simulink model "FFM_Punch"  (R2017a)
settings: Solver=ode3  StartTime=0.0  StopTime=timesteps  FixedStep=data.SIM.Ts  RelTol=1e-3  EnableMultiTasking=on
values from neighbouring files (symbols this model uses):
  data =     [dakota_config.mat]
  downshift_map = data.TCU.upshift.veh_spd_default    [Simulation_results.m]
  upshift_map = data.TCU.upshift.veh_spd_default    [Simulation_results.m]
undefined symbols (not defined in the file or in its folder): air_density, Cd, DiscIntNeverNeededParam, fr_crankshaft, fr_speed_values, g, i_FD, ICE, Low_Ratio, M_Eng_Max, M_Eng_Max_Max, M_Eng_Max_Rpm, mt2m_f, mu_Roll_C0, mu_Roll_C1, mu_Roll_C2, Mv, n_Idle_Eng, Overdrive_Ratio, Re, S_eff_drag, Ts
(part 7 of 15)

== system FFM_Punch/Driver Interface/Driver Model-_old/Rolling Resistance ==
  v_Ref : Inport
  Fcn1 : Fcn  Expr=u(1)*(u(2)+u(3)*u(8)+u(4)*u(8)*u(8)+u(5)*u(8)*u(8)*u(8)+u(6)*u(8)*u(8)*u(8)*u(8)+u(7)*u(8)*u(8)*u(8)*u(8)*u(8))
  Lookup Table : Lookup  InputValues=[-1e3 -1 0 1 1e3 ]  Table=[1 1 0 -1 -1]  LookUpMeth=Interpolation-Use End Values
  Mux1 : Mux  Inputs=8
  Product : Product  RndMeth=Zero
  Roll_res_coeff_C2 : Constant  Value=Mv*g
  Roll_res_coeff_C3 : Constant  Value=mu_Roll_C0
  Roll_res_coeff_C4 : Constant  Value=mu_Roll_C1
  Roll_res_coeff_C5 : Constant  Value=mu_Roll_C2
  Roll_res_coeff_C6 : Constant  Value=0
  kph2m/sec : Gain  Gain=1/3.6  OutDataTypeStr=Inherit: Inherit via back propagation  ParamDataTypeStr=Inherit: Same as input
  mu_Roll_C4 : Constant  Value=0
  mu_Roll_C5 : Constant  Value=0
  radius tyre : Gain  Gain=-Re  OutDataTypeStr=Inherit: Inherit via back propagation  ParamDataTypeStr=Inherit: Same as input
  M_RollingRes : Outport
  wires:
  mu_Roll_C5/1 -> Mux1/7
  kph2m/sec/1 -> Mux1/8
  mu_Roll_C4/1 -> Mux1/6
  Roll_res_coeff_C6/1 -> Mux1/5
  Roll_res_coeff_C5/1 -> Mux1/4
  Product/1 -> M_RollingRes/1
  v_Ref/1 -> kph2m/sec/1, Lookup Table/1
  radius tyre/1 -> Product/1
  Roll_res_coeff_C2/1 -> Mux1/1
  Fcn1/1 -> radius tyre/1
  Roll_res_coeff_C4/1 -> Mux1/3
  Roll_res_coeff_C3/1 -> Mux1/2
  Mux1/1 -> Fcn1/1
  Lookup Table/1 -> Product/2

== system FFM_Punch/Driver Interface/Driver Model-_old/Signed square ==
  note: Air Density
  Vehicle Speed : Inport
  Drag Coefficient : Gain  Gain=Cd  OutDataTypeStr=Inherit: Inherit via back propagation  ParamDataTypeStr=Inherit: Same as input
  Frontal Area : Gain  Gain=S_eff_drag  OutDataTypeStr=Inherit: Inherit via back propagation  ParamDataTypeStr=Inherit: Same as input
  Gain3 : Gain  Gain=0.5
  Product : Product  Inputs=3  RndMeth=Zero
  Sign : Signum  ZeroCross=off
  rho : Gain  Gain=air_density
  Aerodynamic Drag Force : Outport
  wires:
  Sign/1 -> Product/3
  Product/1 -> rho/1
  Gain3/1 -> Aerodynamic Drag Force/1
  Frontal Area/1 -> Gain3/1
  Drag Coefficient/1 -> Frontal Area/1
  rho/1 -> Drag Coefficient/1
  Vehicle Speed/1 -> Product/1, Product/2, Sign/1

== system FFM_Punch/Vehicle/Subsystem/Rolling Resistance ==
  v_veh : Inport
  Abs : Abs
  Constant : Constant  Tag=Controls_Lib  Description=constant  Value=Value  OutMin=OutMin  OutMax=OutMax  OutDataTypeStr=Inherit: Inherit via back propagation  SampleTime=SampleTime  FramePeriod=FramePeriod  mask(Constant){Value=1, VectorParams1D=on, SampleTime=-1, FramePeriod=inf, OutMin=[], OutMax=[], OutDataTypeStr=Inherit: Inherit via back propagation, LockScale=off}
      mask prompts: Value "Simulink:blkprm_prompts:ConstConstValue"; VectorParams1D "Simulink:blkprm_prompts:AllSrcsVector1D"; SampleTime "Simulink:blkprm_prompts:AllSrcBlksSampleTime"; FramePeriod "Simulink:blkprm_prompts:AllSrcBlksFramePeriod"; OutMin "Simulink:blkprm_prompts:OutputDesignMin"; OutMax "Simulink:blkprm_prompts:OutputDesignMax"; OutDataTypeStr "Simulink:blkprm_prompts:OUTPUT_UNIFIEDDATATYPE"; LockScale "Simulink:blkprm_prompts:LockScale"
      mask help: Output the constant specified by the 'Constant value' parameter.
      mask Help: web([fileparts(which('Lib_built')) filesep 'hlp' filesep 'lib_constant' '.html'], '-helpbrowser')
      mask TypeOptions Value: Value
      mask TypeOptions VectorParams1D: VectorParams1D
      mask TypeOptions SampleTime: SampleTime
      mask TypeOptions FramePeriod: FramePeriod
      mask TypeOptions OutMin: OutMin
      mask TypeOptions OutMax: OutMax
      mask TypeOptions OutDataTypeStr: OutDataTypeStr
      mask TypeOptions LockScale: LockScale
      mask DialogControl ParameterTabVar0 Prompt: Main
      mask Display: disp(get_param(gcb,'Value'))
  Constant1 : Constant  Tag=Controls_Lib  Description=constant  Value=Value  OutMin=OutMin  OutMax=OutMax  OutDataTypeStr=Inherit: Inherit via back propagation  SampleTime=SampleTime  FramePeriod=FramePeriod  mask(Constant){Value=0, VectorParams1D=on, SampleTime=-1, FramePeriod=inf, OutMin=[], OutMax=[], OutDataTypeStr=Inherit: Inherit via back propagation, LockScale=off}
      mask prompts: Value "Simulink:blkprm_prompts:ConstConstValue"; VectorParams1D "Simulink:blkprm_prompts:AllSrcsVector1D"; SampleTime "Simulink:blkprm_prompts:AllSrcBlksSampleTime"; FramePeriod "Simulink:blkprm_prompts:AllSrcBlksFramePeriod"; OutMin "Simulink:blkprm_prompts:OutputDesignMin"; OutMax "Simulink:blkprm_prompts:OutputDesignMax"; OutDataTypeStr "Simulink:blkprm_prompts:OUTPUT_UNIFIEDDATATYPE"; LockScale "Simulink:blkprm_prompts:LockScale"
      mask help: Output the constant specified by the 'Constant value' parameter.
      mask Help: web([fileparts(which('Lib_built')) filesep 'hlp' filesep 'lib_constant' '.html'], '-helpbrowser')
      mask TypeOptions Value: Value
      mask TypeOptions VectorParams1D: VectorParams1D
      mask TypeOptions SampleTime: SampleTime
      mask TypeOptions FramePeriod: FramePeriod
      mask TypeOptions OutMin: OutMin
      mask TypeOptions OutMax: OutMax
      mask TypeOptions OutDataTypeStr: OutDataTypeStr
      mask TypeOptions LockScale: LockScale
      mask DialogControl ParameterTabVar0 Prompt: Main
      mask Display: disp(get_param(gcb,'Value'))
  Convert : DataTypeConversion  Tag=Controls_Lib  Description=Convert  OutMin=OutMin  OutMax=OutMax  RndMeth=Round  SampleTime=SampleTime  SaturateOnIntegerOverflow=on  mask(Datatype conversion){ConvertRealWorld=Real World Value (RWV), SampleTime=-1, OutMin=[], OutMax=[], OutDataTypeStr=Inherit: Inherit via back propagation, LockScale=off, RndMeth=Round, SaturateOnIntegerOverflow=on}
      mask prompts: ConvertRealWorld "Input and output to have equal:"; SampleTime "Sample time (-1 for inherited):"; OutMin "Output minimum:"; OutMax "Output maximum:"; OutDataTypeStr "Output data type:"; LockScale "Lock output data type setting against changes by the fixed-point tools"; RndMeth "Integer rounding mode:"; SaturateOnIntegerOverflow "Saturate on integer overflow"
      mask help: Convert the input to the data type and scaling of the output.
      mask Help: web([fileparts(which('Lib_built')) filesep 'hlp' filesep 'lib_DataTypeConv' '.html'], '-helpbrowser')
      mask TypeOptions ConvertRealWorld: ConvertRealWorld
      mask TypeOptions SampleTime: SampleTime
      mask TypeOptions OutMin: OutMin
      mask TypeOptions OutMax: OutMax
      mask TypeOptions OutDataTypeStr: OutDataTypeStr
      mask TypeOptions LockScale: LockScale
      mask TypeOptions RndMeth: RndMeth
      mask TypeOptions SaturateOnIntegerOverflow: SaturateOnIntegerOverflow
  Fcn : Fcn  Expr=u(1)*(u(2)+u(3)*u(8)+u(4)*u(8)*u(8)+u(5)*u(8)*u(8)*u(8)+u(6)*u(8)*u(8)*u(8)*u(8)+u(7)*u(8)*u(8)*u(8)*u(8)*u(8))
  Mux1 : Mux  Inputs=8
  Roll_res_coeff_C0 : Constant  Value=data.VEH.mu_Roll_C0
  Roll_res_coeff_C1 : Constant  Value=data.VEH.mu_Roll_C1
  Roll_res_coeff_C2 : Constant  Value=data.VEH.mu_Roll_C2
  Roll_res_coeff_C3 : Constant  Value=data.VEH.mu_Roll_C3
  Switch : Switch  Criteria=u2 > Threshold  Threshold=eps
  "Weight Vehicle " : Gain  Gain=data.VEH.Mv*data.VEH.g  OutDataTypeStr=Inherit: Inherit via back propagation  ParamDataTypeStr=Inherit: Same as input
  mu_Roll_C4 : Constant  Value=data.VEH.mu_Roll_C4
  mu_Roll_C5 : Constant  Value=data.VEH.mu_Roll_C5
  F_RR : Outport  Tag=Controls_Lib  Description=Out  InitialOutput=0
  wires:
  Abs/1 -> Mux1/8
  mu_Roll_C5/1 -> Mux1/7
  mu_Roll_C4/1 -> Mux1/6
  Roll_res_coeff_C3/1 -> Mux1/5
  Roll_res_coeff_C2/1 -> Mux1/4
  v_veh/1 -> Switch/2, Abs/1
  Roll_res_coeff_C1/1 -> Mux1/3
  Roll_res_coeff_C0/1 -> Mux1/2
  Mux1/1 -> Fcn/1
  "Weight Vehicle "/1 -> Mux1/1
  Constant/1 -> "Weight Vehicle "/1
  Fcn/1 -> Convert/1
  Constant1/1 -> Switch/3
  Switch/1 -> F_RR/1
  Convert/1 -> Switch/1

== system FFM_Punch/Vehicle/Subsystem/Signed square ==
  note: Air Density
  Vehicle Speed : Inport
  Convert : DataTypeConversion  Tag=Controls_Lib  Description=Convert  OutMin=OutMin  OutMax=OutMax  RndMeth=Round  SampleTime=SampleTime  SaturateOnIntegerOverflow=on  mask(Datatype conversion){ConvertRealWorld=Real World Value (RWV), SampleTime=-1, OutMin=[], OutMax=[], OutDataTypeStr=Inherit: Inherit via back propagation, LockScale=off, RndMeth=Round, SaturateOnIntegerOverflow=on}
      mask prompts: ConvertRealWorld "Input and output to have equal:"; SampleTime "Sample time (-1 for inherited):"; OutMin "Output minimum:"; OutMax "Output maximum:"; OutDataTypeStr "Output data type:"; LockScale "Lock output data type setting against changes by the fixed-point tools"; RndMeth "Integer rounding mode:"; SaturateOnIntegerOverflow "Saturate on integer overflow"
      mask help: Convert the input to the data type and scaling of the output.
      mask Help: web([fileparts(which('Lib_built')) filesep 'hlp' filesep 'lib_DataTypeConv' '.html'], '-helpbrowser')
      mask TypeOptions ConvertRealWorld: ConvertRealWorld
      mask TypeOptions SampleTime: SampleTime
      mask TypeOptions OutMin: OutMin
      mask TypeOptions OutMax: OutMax
      mask TypeOptions OutDataTypeStr: OutDataTypeStr
      mask TypeOptions LockScale: LockScale
      mask TypeOptions RndMeth: RndMeth
      mask TypeOptions SaturateOnIntegerOverflow: SaturateOnIntegerOverflow
  Drag Coefficient : Gain  Gain=data.VEH.Cd  OutDataTypeStr=Inherit: Inherit via back propagation  ParamDataTypeStr=Inherit: Same as input
  Frontal Area : Gain  Gain=data.VEH.S_eff_drag  OutDataTypeStr=Inherit: Inherit via back propagation  ParamDataTypeStr=Inherit: Same as input
  Gain3 : Gain  Gain=0.5
  Product : Product  RndMeth=Zero
  Product1 : Product  RndMeth=Zero
  Sign : Signum  ZeroCross=off
  rho : Gain  Gain=data.VEH.air_density
  Aerodynamic Drag Force : Outport
  wires:
  Sign/1 -> Product/2
  Frontal Area/1 -> Gain3/1
  Drag Coefficient/1 -> Frontal Area/1
  rho/1 -> Drag Coefficient/1
  Product/1 -> rho/1
  Vehicle Speed/1 -> Product1/2, Product1/1, Sign/1
  Product1/1 -> Product/1
  Gain3/1 -> Convert/1
  Convert/1 -> Aerodynamic Drag Force/1

== system FFM_Punch/Controller/F02_03_03_05_Raw_Gear_Target_Auto_Mode/F02_03_03_05_09_Final_Raw_Gear_Target_Auto_Mode/TurnOnDelay1 ==
  b_Input : Inport  Tag=Controls_Lib  Description=Inp  OutDataTypeStr=boolean  Interpolate=off
  Tdly : Inport  Tag=Controls_Lib  Description=Inp  Port=2  OutDataTypeStr=single  Interpolate=off
  Constant2 : Constant  Tag=Controls_Lib  Description=constant  Value=Value  OutMin=OutMin  OutMax=OutMax  OutDataTypeStr=boolean  SampleTime=SampleTime  FramePeriod=FramePeriod  mask(Constant){Value=0, VectorParams1D=on, SampleTime=-1, FramePeriod=inf, OutMin=[], OutMax=[], OutDataTypeStr=boolean, LockScale=off}
      mask prompts: Value "Simulink:blkprm_prompts:ConstConstValue"; VectorParams1D "Simulink:blkprm_prompts:AllSrcsVector1D"; SampleTime "Simulink:blkprm_prompts:AllSrcBlksSampleTime"; FramePeriod "Simulink:blkprm_prompts:AllSrcBlksFramePeriod"; OutMin "Simulink:blkprm_prompts:OutputDesignMin"; OutMax "Simulink:blkprm_prompts:OutputDesignMax"; OutDataTypeStr "Simulink:blkprm_prompts:OUTPUT_UNIFIEDDATATYPE"; LockScale "Simulink:blkprm_prompts:LockScale"
      mask help: Output the constant specified by the 'Constant value' parameter.
      mask Help: web([fileparts(which('Lib_built')) filesep 'hlp' filesep 'lib_constant' '.html'], '-helpbrowser')
      mask TypeOptions Value: Value
      mask TypeOptions VectorParams1D: VectorParams1D
      mask TypeOptions SampleTime: SampleTime
      mask TypeOptions FramePeriod: FramePeriod
      mask TypeOptions OutMin: OutMin
      mask TypeOptions OutMax: OutMax
      mask TypeOptions OutDataTypeStr: OutDataTypeStr
      mask TypeOptions LockScale: LockScale
      mask DialogControl ParameterTabVar0 Prompt: Main
      mask Display: disp(get_param(gcb,'Value'))
  Logic : Logic  Tag=Controls_Lib  Description=Logic  Operator=NOT  Inputs=Inputs  OutDataTypeStr=boolean  SampleTime=SampleTime  mask(Logic){Operator=NOT, Inputs=2, IconShape=rectangular, SampleTime=-1, AllPortsSameDT=on, OutDataTypeStr=boolean}
      mask prompts: Inputs "Number of input ports:"; IconShape "Icon shape:"; SampleTime "Sample time (-1 for inherited):"; AllPortsSameDT "Require all inputs and output to have the same data type"; OutDataTypeStr "Output data type:"
      mask help: Logical operators. For a single input, operators are applied across the input vector. For multiple inputs, operators are applied across the inputs.
      mask Help: web([fileparts(which('Lib_built')) filesep 'hlp' filesep 'lib_Logic' '.html'], '-helpbrowser')
      mask TypeOptions Operator: Operator
      mask TypeOptions Inputs: Inputs
      mask TypeOptions IconShape: IconShape
      mask TypeOptions SampleTime: SampleTime
      mask TypeOptions AllPortsSameDT: AllPortsSameDT
      mask TypeOptions OutDataTypeStr: OutDataTypeStr
  Logic1 : Logic  Tag=Controls_Lib  Description=Logic  Operator=NOT  Inputs=Inputs  OutDataTypeStr=boolean  SampleTime=SampleTime  mask(Logic){Operator=NOT, Inputs=2, IconShape=rectangular, SampleTime=-1, AllPortsSameDT=on, OutDataTypeStr=boolean}
      mask prompts: Inputs "Number of input ports:"; IconShape "Icon shape:"; SampleTime "Sample time (-1 for inherited):"; AllPortsSameDT "Require all inputs and output to have the same data type"; OutDataTypeStr "Output data type:"
      mask help: Logical operators. For a single input, operators are applied across the input vector. For multiple inputs, operators are applied across the inputs.
      mask Help: web([fileparts(which('Lib_built')) filesep 'hlp' filesep 'lib_Logic' '.html'], '-helpbrowser')
      mask TypeOptions Operator: Operator
      mask TypeOptions Inputs: Inputs
      mask TypeOptions IconShape: IconShape
      mask TypeOptions SampleTime: SampleTime
      mask TypeOptions AllPortsSameDT: AllPortsSameDT
      mask TypeOptions OutDataTypeStr: OutDataTypeStr
  Rising_Edge_DetectChange1 : Subsystem  Tag=Controls_Lib  Description=DetectChange  mask(Rising_Edge_Detect_change){}
      mask help:
      | Rising Edge Detect change block will detect the change in input signal.The block output will be true for one sample when input chnage from false to true.
      |
      | Note: Input and initial conditions must always be a boolean. Initial condition is used to enable or disable the edge detection at the very first instant. No Edge will be detected at the first instant if the Initial condition is set to be equal to the Input signal.
      mask init:
      | x1=[1 2 2 4 4 5];
      | y1=[7 7 9 9 9 9];
      | x2=[1 2 2 4 4 5];
      | y2=[0 0 0 0 0 0];
      mask Help: web([fileparts(which('Lib_discontious')) filesep 'hlp' filesep 'lib_DetectChange.html'], '-helpbrowser')
      mask Display: plot(x1,y1);plot(x2,y2);
  Terminator1 : Terminator
      settings: Tag=Controls_Lib  Description=Terminator
  Timer : Subsystem  Tag=Controls_Lib  Description=Timer  mask(Timer){}
      mask help:
      | This block counts down from TT to 0 (zero) when a falling edge is detected in the the 'Res' port. When the timer is active and 'Res' is FALSE, 'TL' specifies the time left to reach 0(zero). When 'Res' is TRUE, TL=TT. The output 'Busy' is TRUE when 'Res' TRUE or the timer is actively counting(i.e until 'TL' is 0(zero) ).
      |
      | Ports:
      | TT - Target Time [sec] [Single]
      | Res - Reset [-] [Boolean]
      | Busy - Busy status [-] [Boolean]
      | TL - Time Left [Sec] [Single]
      |
      | Input Guidelines:
      |
      | 1.The input 'TT' must always be a positive non-zero number.
      | 2.The input 'TT' must be a multiple of the fundamental sample time of the block.
      settings: RTWSystemCode=Inline
      mask Help: web([fileparts(which('Lib_math_logic')) filesep 'hlp' filesep 'lib_Timer.html'], '-helpbrowser')
      mask Display:
      | disp('Timer');
      | port_label('Input',1,'Res');
      | port_label('Input',2,'TT [s]');
      | port_label('Output',1,'Busy');
      | port_label('Output',2,'TL [s]');
  b_Output : Outport  OutDataTypeStr=boolean  OutputWhenDisabled=reset  InitialOutput=0
  wires:
  Timer/2(TL) -> Terminator1/1
  Timer/1(Busy) -> Logic1/1
  Logic/1 -> Timer/1(Res)
  b_Input/1 -> Logic/1
  Tdly/1 -> Timer/2(TT)
  Logic1/1 -> Rising_Edge_DetectChange1/1(b_Input)
  Rising_Edge_DetectChange1/1(b_Output) -> b_Output/1
  Constant2/1 -> Rising_Edge_DetectChange1/2(b_InitialValue)

== system FFM_Punch/Controller/F02_03_03_05_Raw_Gear_Target_Auto_Mode/F02_03_03_05_09_Final_Raw_Gear_Target_Auto_Mode/TurnOnDelay2 ==
  b_Input : Inport  Tag=Controls_Lib  Description=Inp  OutDataTypeStr=boolean  Interpolate=off
  Tdly : Inport  Tag=Controls_Lib  Description=Inp  Port=2  OutDataTypeStr=single  Interpolate=off
  Constant2 : Constant  Tag=Controls_Lib  Description=constant  Value=Value  OutMin=OutMin  OutMax=OutMax  OutDataTypeStr=boolean  SampleTime=SampleTime  FramePeriod=FramePeriod  mask(Constant){Value=0, VectorParams1D=on, SampleTime=-1, FramePeriod=inf, OutMin=[], OutMax=[], OutDataTypeStr=boolean, LockScale=off}
      mask prompts: Value "Simulink:blkprm_prompts:ConstConstValue"; VectorParams1D "Simulink:blkprm_prompts:AllSrcsVector1D"; SampleTime "Simulink:blkprm_prompts:AllSrcBlksSampleTime"; FramePeriod "Simulink:blkprm_prompts:AllSrcBlksFramePeriod"; OutMin "Simulink:blkprm_prompts:OutputDesignMin"; OutMax "Simulink:blkprm_prompts:OutputDesignMax"; OutDataTypeStr "Simulink:blkprm_prompts:OUTPUT_UNIFIEDDATATYPE"; LockScale "Simulink:blkprm_prompts:LockScale"
      mask help: Output the constant specified by the 'Constant value' parameter.
      mask Help: web([fileparts(which('Lib_built')) filesep 'hlp' filesep 'lib_constant' '.html'], '-helpbrowser')
      mask TypeOptions Value: Value
      mask TypeOptions VectorParams1D: VectorParams1D
      mask TypeOptions SampleTime: SampleTime
      mask TypeOptions FramePeriod: FramePeriod
      mask TypeOptions OutMin: OutMin
      mask TypeOptions OutMax: OutMax
      mask TypeOptions OutDataTypeStr: OutDataTypeStr
      mask TypeOptions LockScale: LockScale
      mask DialogControl ParameterTabVar0 Prompt: Main
      mask Display: disp(get_param(gcb,'Value'))
  Logic : Logic  Tag=Controls_Lib  Description=Logic  Operator=NOT  Inputs=Inputs  OutDataTypeStr=boolean  SampleTime=SampleTime  mask(Logic){Operator=NOT, Inputs=2, IconShape=rectangular, SampleTime=-1, AllPortsSameDT=on, OutDataTypeStr=boolean}
      mask prompts: Inputs "Number of input ports:"; IconShape "Icon shape:"; SampleTime "Sample time (-1 for inherited):"; AllPortsSameDT "Require all inputs and output to have the same data type"; OutDataTypeStr "Output data type:"
      mask help: Logical operators. For a single input, operators are applied across the input vector. For multiple inputs, operators are applied across the inputs.
      mask Help: web([fileparts(which('Lib_built')) filesep 'hlp' filesep 'lib_Logic' '.html'], '-helpbrowser')
      mask TypeOptions Operator: Operator
      mask TypeOptions Inputs: Inputs
      mask TypeOptions IconShape: IconShape
      mask TypeOptions SampleTime: SampleTime
      mask TypeOptions AllPortsSameDT: AllPortsSameDT
      mask TypeOptions OutDataTypeStr: OutDataTypeStr
  Logic1 : Logic  Tag=Controls_Lib  Description=Logic  Operator=NOT  Inputs=Inputs  OutDataTypeStr=boolean  SampleTime=SampleTime  mask(Logic){Operator=NOT, Inputs=2, IconShape=rectangular, SampleTime=-1, AllPortsSameDT=on, OutDataTypeStr=boolean}
      mask prompts: Inputs "Number of input ports:"; IconShape "Icon shape:"; SampleTime "Sample time (-1 for inherited):"; AllPortsSameDT "Require all inputs and output to have the same data type"; OutDataTypeStr "Output data type:"
      mask help: Logical operators. For a single input, operators are applied across the input vector. For multiple inputs, operators are applied across the inputs.
      mask Help: web([fileparts(which('Lib_built')) filesep 'hlp' filesep 'lib_Logic' '.html'], '-helpbrowser')
      mask TypeOptions Operator: Operator
      mask TypeOptions Inputs: Inputs
      mask TypeOptions IconShape: IconShape
      mask TypeOptions SampleTime: SampleTime
      mask TypeOptions AllPortsSameDT: AllPortsSameDT
      mask TypeOptions OutDataTypeStr: OutDataTypeStr
  Rising_Edge_DetectChange1 : Subsystem  Tag=Controls_Lib  Description=DetectChange  mask(Rising_Edge_Detect_change){}
      mask help:
      | Rising Edge Detect change block will detect the change in input signal.The block output will be true for one sample when input chnage from false to true.
      |
      | Note: Input and initial conditions must always be a boolean. Initial condition is used to enable or disable the edge detection at the very first instant. No Edge will be detected at the first instant if the Initial condition is set to be equal to the Input signal.
      mask init:
      | x1=[1 2 2 4 4 5];
      | y1=[7 7 9 9 9 9];
      | x2=[1 2 2 4 4 5];
      | y2=[0 0 0 0 0 0];
      mask Help: web([fileparts(which('Lib_discontious')) filesep 'hlp' filesep 'lib_DetectChange.html'], '-helpbrowser')
      mask Display: plot(x1,y1);plot(x2,y2);
  Terminator1 : Terminator
      settings: Tag=Controls_Lib  Description=Terminator
  Timer : Subsystem  Tag=Controls_Lib  Description=Timer  mask(Timer){}
      mask help:
      | This block counts down from TT to 0 (zero) when a falling edge is detected in the the 'Res' port. When the timer is active and 'Res' is FALSE, 'TL' specifies the time left to reach 0(zero). When 'Res' is TRUE, TL=TT. The output 'Busy' is TRUE when 'Res' TRUE or the timer is actively counting(i.e until 'TL' is 0(zero) ).
      |
      | Ports:
      | TT - Target Time [sec] [Single]
      | Res - Reset [-] [Boolean]
      | Busy - Busy status [-] [Boolean]
      | TL - Time Left [Sec] [Single]
      |
      | Input Guidelines:
      |
      | 1.The input 'TT' must always be a positive non-zero number.
      | 2.The input 'TT' must be a multiple of the fundamental sample time of the block.
      settings: RTWSystemCode=Inline
      mask Help: web([fileparts(which('Lib_math_logic')) filesep 'hlp' filesep 'lib_Timer.html'], '-helpbrowser')
      mask Display:
      | disp('Timer');
      | port_label('Input',1,'Res');
      | port_label('Input',2,'TT [s]');
      | port_label('Output',1,'Busy');
      | port_label('Output',2,'TL [s]');
  b_Output : Outport  OutDataTypeStr=boolean  OutputWhenDisabled=reset  InitialOutput=0
  wires:
  Constant2/1 -> Rising_Edge_DetectChange1/2(b_InitialValue)
  Rising_Edge_DetectChange1/1(b_Output) -> b_Output/1
  Logic1/1 -> Rising_Edge_DetectChange1/1(b_Input)
  Tdly/1 -> Timer/2(TT)
  b_Input/1 -> Logic/1
  Logic/1 -> Timer/1(Res)
  Timer/1(Busy) -> Logic1/1
  Timer/2(TL) -> Terminator1/1

== system FFM_Punch/Driver Interface/Driver Mode_pedalbased/Driver PID Error Calculation and ffwd/FirstOrderDerivative1 ==
  Input : Inport  Tag=Controls_Lib  Description=Inp  OutDataTypeStr=single  Interpolate=off
  AddSub2 : Sum  Tag=Controls_Lib  Description=AddSub  Inputs=+-  CollapseDim=CollapseDim  AccumDataTypeStr=single  OutMin=OutMin  OutMax=OutMax  OutDataTypeStr=single  RndMeth=Nearest  SampleTime=SampleTime  InputSameDT=on  mask(AddSub){IconShape=rectangular, Inputs=+-, CollapseMode=All dimensions, CollapseDim=1, SampleTime=-1, InputSameDT=on, AccumDataTypeStr=single, OutMin=[], OutMax=[], OutDataTypeStr=single, LockScale=off, RndMeth=Nearest, SaturateOnIntegerOverflow=off}
      mask prompts: IconShape "Icon shape:"; Inputs "List of signs:"; CollapseMode "Sum over:"; CollapseDim "Dimension:"; SampleTime "Sample time (-1 for inherited):"; InputSameDT "Require all inputs to have the same data type"; AccumDataTypeStr "Accumulator data type:"; OutMin "Output minimum:"; OutMax "Output maximum:"; OutDataTypeStr "Output data type:"; LockScale "Lock data type settings against changes by the fixed-point tools"; RndMeth "Integer rounding mode:"; SaturateOnIntegerOverflow "Saturate on integer overflow"
      mask help:
      | Add or subtract inputs.  Specify one of the following:
      | a) string containing + or - for each input port, | for spacer between ports (e.g. ++|-|++)
      | b) scalar, >= 1, specifies the number of input ports to be summed.
      | When there is only one input port, add or subtract elements over all dimensions or one specified dimension
      mask Help: web([fileparts(which('Lib_built')) filesep 'hlp' filesep 'lib_AddSub' '.html'], '-helpbrowser')
      mask TypeOptions IconShape: IconShape
      mask TypeOptions Inputs: Inputs
      mask TypeOptions CollapseMode: CollapseMode
      mask TypeOptions CollapseDim: CollapseDim
      mask TypeOptions SampleTime: SampleTime
      mask TypeOptions InputSameDT: InputSameDT
      mask TypeOptions AccumDataTypeStr: AccumDataTypeStr
      mask TypeOptions OutMin: OutMin
      mask TypeOptions OutMax: OutMax
      mask TypeOptions OutDataTypeStr: OutDataTypeStr
      mask TypeOptions LockScale: LockScale
      mask TypeOptions RndMeth: RndMeth
      mask TypeOptions SaturateOnIntegerOverflow: SaturateOnIntegerOverflow
  Delay1 : Delay  Tag=Controls_Lib  Description=VariableDelay  DelayLength=DelayLength  DelayLengthUpperLimit=DelayLengthUpperLimit  InitialConditionSource=Input port  InitialCondition=InitialCondition  SampleTime=SampleTime  mask(Delay){DelayLengthSource=Dialog, DelayLength=1, DelayLengthUpperLimit=100, InitialConditionSource=Input port, InitialCondition=0.0, ExternalReset=None, PreventDirectFeedthrough=off, DiagnosticForOutOfRangeDelayLength=None, RemoveProtectionDelayLength=off, InputProcessing=Elements as channels (sample based), UseCircularBuffer=off, SampleTime=-1, StateName=, StateMustResolveToSignalObject=off, CodeGenStateStorageClass=Auto, CodeGenStateStorageTypeQualifier=}
      mask prompts: DelayLengthSource "Delay length source:"; DelayLength "Delay length:"; DelayLengthUpperLimit "Delay upper limit:"; InitialConditionSource "Initial condition source:"; InitialCondition "Initial condition:"; ExternalReset "External reset:"; PreventDirectFeedthrough "Prevent direct feedthrough by increasing delay length to lower limit"; DiagnosticForOutOfRangeDelayLength "Diagnostic for out-of-range delay length:"; RemoveProtectionDelayLength "Remove protection against out-of-range delay length in generated code"; InputProcessing "Input processing:"; UseCircularBuffer "Use circular buffer for state"; SampleTime "Sample time (-1 for inherited):"; StateName "State name:"; StateMustResolveToSignalObject "State name must resolve to Simulink signal object"; CodeGenStateStorageClass "Code generation storage class:"; CodeGenStateStorageTypeQualifier "Code generation storage type qualifier:"
      mask help: Delay input by a fixed or variable number of samples. The initial output of the delay block is specified by the external input x0.
      settings: InputPortMap=u0,p4
      mask Help: web([fileparts(which('Lib_discrete')) filesep 'hlp' filesep 'lib_Delay.html'], '-helpbrowser')
      mask TypeOptions DelayLengthSource: DelayLengthSource
      mask TypeOptions DelayLength: DelayLength
      mask TypeOptions DelayLengthUpperLimit: DelayLengthUpperLimit
      mask TypeOptions InitialConditionSource: InitialConditionSource
      mask TypeOptions InitialCondition: InitialCondition
      mask TypeOptions ExternalReset: ExternalReset
      mask TypeOptions PreventDirectFeedthrough: PreventDirectFeedthrough
      mask TypeOptions DiagnosticForOutOfRangeDelayLength: DiagnosticForOutOfRangeDelayLength
      mask TypeOptions RemoveProtectionDelayLength: RemoveProtectionDelayLength
      mask TypeOptions InputProcessing: InputProcessing
      mask TypeOptions UseCircularBuffer: UseCircularBuffer
      mask TypeOptions SampleTime: SampleTime
      mask TypeOptions StateName: StateName
      mask TypeOptions StateMustResolveToSignalObject: StateMustResolveToSignalObject
      mask TypeOptions CodeGenStateStorageClass: CodeGenStateStorageClass
      mask TypeOptions CodeGenStateStorageTypeQualifier: CodeGenStateStorageTypeQualifier
  MulDiv : Product  Tag=Controls_Lib  Description=MulDiv  Inputs=**  CollapseDim=CollapseDim  OutMin=OutMin  OutMax=OutMax  OutDataTypeStr=single  SampleTime=SampleTime  InputSameDT=on  mask(MulDiv){Inputs=**, Multiplication=Element-wise(.*), CollapseMode=All dimensions, CollapseDim=1, SampleTime=-1, InputSameDT=on, OutMin=[], OutMax=[], OutDataTypeStr=single, LockScale=off, RndMeth=Floor, SaturateOnIntegerOverflow=off}
      mask prompts: Inputs "Number of inputs:"; CollapseMode "Multiply over:"; CollapseDim "Dimension:"; SampleTime "Sample time (-1 for inherited):"; InputSameDT "Require all inputs to have the same data type"; OutMin "Output minimum:"; OutMax "Output maximum:"; OutDataTypeStr "Output data type:"; LockScale "Lock output data type setting against changes by the fixed-point tools"; RndMeth "Integer rounding mode:"; SaturateOnIntegerOverflow "Saturate on integer overflow"
      mask help:
      | Multiply or divide inputs element-wise. Specify one of the following:
      |  a) * or / for each input port. For example, **/* performs the operation 'u1*u2/u3*u4'.
      |  b) scalar specifies the number of input ports to be multiplied.
      | If there is only one input port and the Multiplication parameter is set to Element-wise(.*), a single * or / collapses the input signal using the specified operation.
      mask Help: web([fileparts(which('Lib_built')) filesep 'hlp' filesep 'lib_MulDiv' '.html'], '-helpbrowser')
      mask TypeOptions Inputs: Inputs
      mask TypeOptions Multiplication: Multiplication
      mask TypeOptions CollapseMode: CollapseMode
      mask TypeOptions CollapseDim: CollapseDim
      mask TypeOptions SampleTime: SampleTime
      mask TypeOptions InputSameDT: InputSameDT
      mask TypeOptions OutMin: OutMin
      mask TypeOptions OutMax: OutMax
      mask TypeOptions OutDataTypeStr: OutDataTypeStr
      mask TypeOptions LockScale: LockScale
      mask TypeOptions RndMeth: RndMeth
      mask TypeOptions SaturateOnIntegerOverflow: SaturateOnIntegerOverflow
  TsInverse1 : SampleTimeMath  Tag=Controls_Lib  Description=TsInverse  TsampMathOp=1/Ts Only  weightValue=weightValue  OutDataTypeStr=Inherit: Inherit via back propagation  mask(Sample time block){TsampMathOp=1/Ts Only, weightValue=1, TsampMathImp=Online Calculations, OutDataTypeStr=Inherit: Inherit via back propagation, RndMeth=Floor, SaturateOnIntegerOverflow=off}
      mask prompts: TsampMathOp "Operation:"; weightValue "Weight value:"; TsampMathImp "Implement using:"; OutDataTypeStr "Output data type:"; RndMeth "Integer rounding mode:"; SaturateOnIntegerOverflow "Saturate on integer overflow"
      mask help: 1 divided by the Sample time of the input signal
      mask Help: web([fileparts(which('Lib_built')) filesep 'hlp' filesep 'lib_TsInv' '.html'], '-helpbrowser')
      mask TypeOptions TsampMathOp: TsampMathOp
      mask TypeOptions weightValue: weightValue
      mask TypeOptions TsampMathImp: TsampMathImp
      mask TypeOptions OutDataTypeStr: OutDataTypeStr
      mask TypeOptions RndMeth: RndMeth
      mask TypeOptions SaturateOnIntegerOverflow: SaturateOnIntegerOverflow
  Output : Outport  Tag=Controls_Lib  Description=Out  OutDataTypeStr=single  InitialOutput=0
  wires:
  TsInverse1/1 -> MulDiv/2
  MulDiv/1 -> AddSub2/1, Delay1/2, Delay1/1  "Inputrate"
  Input/1 -> MulDiv/1, TsInverse1/1  "Input"
  AddSub2/1 -> Output/1  "DerivativeOutput"
  Delay1/1 -> AddSub2/2  "PrevInpRate"
